simulink model "test_washing_machine"  (R2024b)
settings: Solver=VariableStepAuto  StartTime=0.0  StopTime=inf  RelTol=1e-3
settings Model: Creator=Dell  LastModifiedBy=Dell

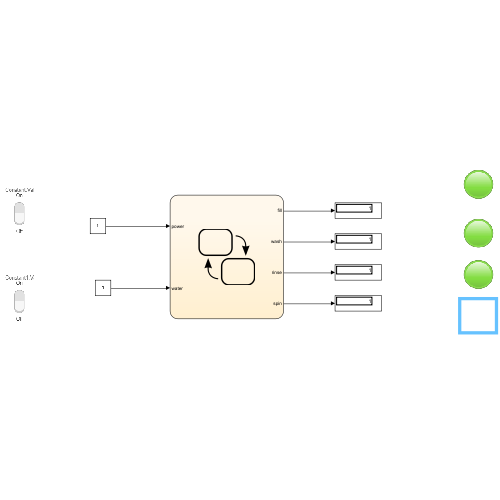
[thumbnail: Simulink's stored preview of the top-level diagram]
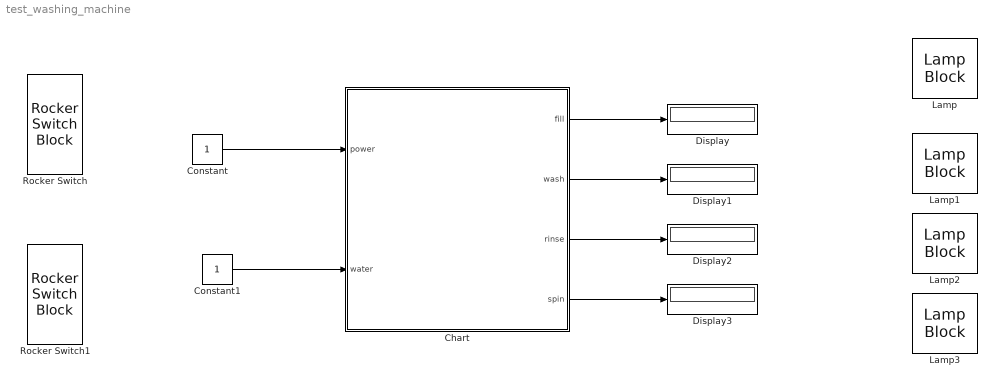
== system test_washing_machine ==
  Chart : Stateflow chart  TreatAsAtomicUnit=on
  Constant : Constant
  Constant1 : Constant
  Display{,1..3} (4 alike) : Display
  Lamp{,1..3} (4 alike) : LampBlock  LabelPosition=Hide
  Rocker Switch : RockerSwitchBlock
      settings: Values={{'Off', 'On'}, [0 1]}
  Rocker Switch1 : RockerSwitchBlock
      settings: Values={{'Off', 'On'}, [0 1]}
  wires:
  Chart/1(fill) -> Display/1
  Chart/2(wash) -> Display1/1
  Chart/3(rinse) -> Display2/1
  Chart/4(spin) -> Display3/1
  Constant/1 -> Chart/1(power)
  Constant1/1 -> Chart/2(water)

== stateflow chart test_washing_machine/Chart ==
  state Idle
    power==0
  state water
    entry:
    water==0
  state fill
    entry:
    fill=1
  state wash
    entry:
    wash=1
  state rinse
    entry:
    rinse=1
  state spin
    entry:
    spin=1
  state end
    entry:
  (default) -> Idle
  Idle -> water : [power==1]
  fill -> wash : [after(10,sec)]
  wash -> rinse : [after(10,sec)]
  water -> fill : [water==1]
  rinse -> spin : [after(10,sec)]
  spin -> end : [after(10,sec)]
  data: fill output; wash output; rinse output; spin output; power input; water input
